simulink model "Q6"  (R2019a)
settings: Solver=VariableStepAuto  StartTime=0.0  StopTime=10.0  RelTol=1e-3
settings Model: Creator=linesLK  LastModifiedBy=linesLK

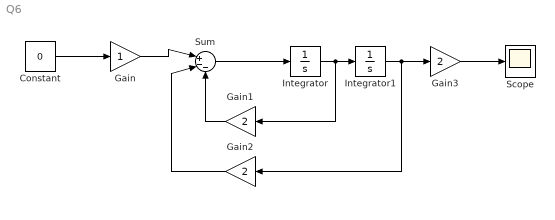
== system Q6 ==
  Constant : Constant  Value=0
  Gain : Gain
  Gain1 : Gain  Gain=2
  Gain2 : Gain  Gain=2
  Gain3 : Gain  Gain=2
  Integrator : Integrator
  Integrator1 : Integrator  InitialCondition=1/2
  Scope : Scope
  Sum : Sum  Inputs=|+--
  wires:
  Constant/1 -> Gain/1
  Gain/1 -> Sum/1
  Sum/1 -> Integrator/1
  Integrator/1 -> Gain1/1, Integrator1/1
  Gain1/1 -> Sum/3
  Gain2/1 -> Sum/2
  Integrator1/1 -> Gain3/1, Gain2/1
  Gain3/1 -> Scope/1
